simulink model "Bandstop"  (R2020a)
settings: Solver=FixedStepDiscrete  StartTime=0.0  StopTime=10.0  RelTol=1e-3
settings Model: Creator=yuzehong  LastModifiedBy=sadamu
settings OptimizationCC: DefaultParameterBehavior=Inlined  UseDivisionForNetSlopeComputation=on  GainParamInheritBuiltInType=on  UseFloatMulNetSlope=on  InlineInvariantSignals=on  OptimizeBlockIOStorage=off  BufferReuse=off  GlobalBufferReuse=off  ExpressionFolding=off  EnableMemcpy=off  PassReuseOutputArgsAs=Individual arguments  LocalBlockOutputs=off  ZeroExternalMemoryAtStartup=off  ZeroInternalMemoryAtStartup=off  NoFixptDivByZeroProtection=on  EfficientFloat2IntCast=on  LifeSpan=1  OptimizeDataStoreBuffers=off  BusAssignmentInplaceUpdate=off  OptimizationLevel=level0  OptimizationCustomize=off  EfficientTunableParamExpr=on
settings DebuggingCC: ParameterTunabilityLossMsg=error  SFMachineParentedDataDiag=error
settings SFSimCC: MATLABDynamicMemAlloc=off  CustomCodeUndefinedFunction=UseInterfaceOnly
settings RTWCC: SystemTargetFile=ert.tlc  TemplateMakefile=ert_default_tmf  GenerateReport=on  LaunchReport=on
settings CodeAppCC: GenerateComments=off  IgnoreCustomStorageClasses=off  OperatorAnnotations=on  SimulinkDataObjDesc=on  SFDataObjDesc=on  CustomSymbolStrGlobalVar=rt$N$M  CustomSymbolStrType=$N$M  CustomSymbolStrFcn=$N$M$F  CustomSymbolStrMacro=$N$M  SimulinkBlockComments=off
settings ERTTargetCC: TargetLangStandard=C99 (ISO)  CodeReplacementLibrary=Intel AVX (Windows)  GenerateSampleERTMain=on  IncludeMdlTerminateFcn=off  CombineSignalStateStructs=on  SuppressErrorStatus=on  SupportAbsoluteTime=off  PurelyIntegerCode=on  SupportNonFinite=off  SupportComplex=off  InlinedParameterPlacement=NonHierarchical  ERTCustomFileTemplate=example_file_process.tlc  ERTFilePackagingFormat=CompactWithDataFile

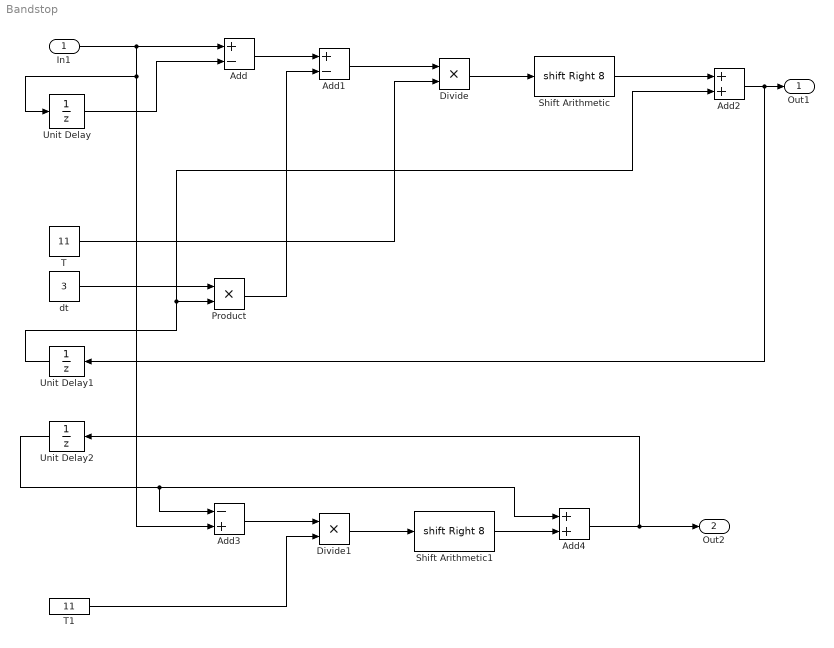
== system Bandstop ==
  In1 : Inport  OutDataTypeStr=int32  PortDimensions=1
  Add : Sum  Inputs=+-
  Add1 : Sum  Inputs=+-
  Add2 : Sum
  Add3 : Sum  Inputs=-+
  Add4 : Sum
  Divide : Product  Inputs=**  OutDataTypeStr=int32
  Divide1 : Product  Inputs=**  OutDataTypeStr=int32  RndMeth=Simplest
  Product : Product  OutDataTypeStr=int32
  Shift Arithmetic : ArithShift  BitShiftNumber=8  BitShiftDirection=Right
  Shift Arithmetic1 : ArithShift  BitShiftNumber=8  BitShiftDirection=Right
  T : Constant  Value=11  OutDataTypeStr=int32  SampleTime=0.1
  T1 : Constant  Value=11  OutDataTypeStr=int32  SampleTime=0.1
  Unit Delay : UnitDelay  SampleTime=-1  HasFrameUpgradeWarning=on
  Unit Delay1 : UnitDelay  SampleTime=-1  HasFrameUpgradeWarning=on
  Unit Delay2 : UnitDelay  SampleTime=-1  HasFrameUpgradeWarning=on
  dt : Constant  Value=3  OutDataTypeStr=int32  SampleTime=0.1
  Out1 : Outport
  Out2 : Outport  Port=2
  wires:
  T/1 -> Divide/2
  Product/1 -> Add1/2
  In1/1 -> Unit Delay/1, Add3/2, Add/1
  Unit Delay1/1 -> Product/2, Add2/2
  Unit Delay/1 -> Add/2
  Shift Arithmetic/1 -> Add2/1
  Add2/1 -> Unit Delay1/1, Out1/1
  Divide/1 -> Shift Arithmetic/1
  Add/1 -> Add1/1
  dt/1 -> Product/1
  Add1/1 -> Divide/1
  Divide1/1 -> Shift Arithmetic1/1
  Shift Arithmetic1/1 -> Add4/2
  Add4/1 -> Out2/1, Unit Delay2/1
  T1/1 -> Divide1/2
  Unit Delay2/1 -> Add4/1, Add3/1
  Add3/1 -> Divide1/1
